simulink model "CW1_Pure_Pursuit_sim"  (R2023a)
settings: Solver=VariableStepAuto  StartTime=0.0  StopTime=Ts  RelTol=1e-3
values from neighbouring files (symbols this model uses):
  L = 3    [CW1_Pure_Pursuit.m]
  ld = 5    [CW1_Pure_Pursuit.m]
  psi_o = 90*rand(1)    [CW1_Pure_Pursuit.m]
  veh_v0 = 8    [CW1_Pure_Pursuit.m]    (also in DrivingScenario_LearnVersion.m)
  X_o = refPose(1,1)    [CW1_Pure_Pursuit.m]
  xRef = refPose(1,:)'    [CW1_Pure_Pursuit.m]
  Y_o = refPose(1,2)    [CW1_Pure_Pursuit.m]
  yRef = refPose(2,:)'    [CW1_Pure_Pursuit.m]
libraries: robotalgslib x1, autolibshared x1
settings Model: Creator=Gabriel  LastModifiedBy=Gabriel

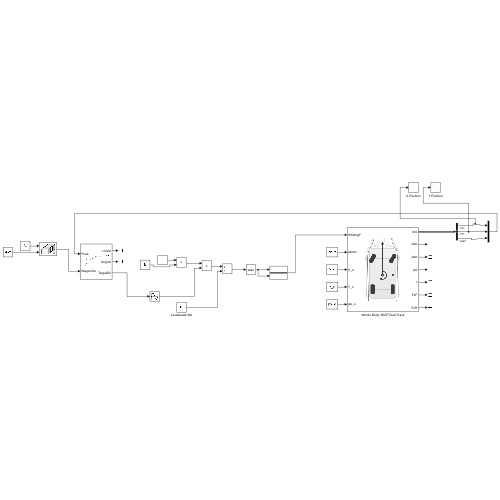
[thumbnail: Simulink's stored preview of the top-level diagram]
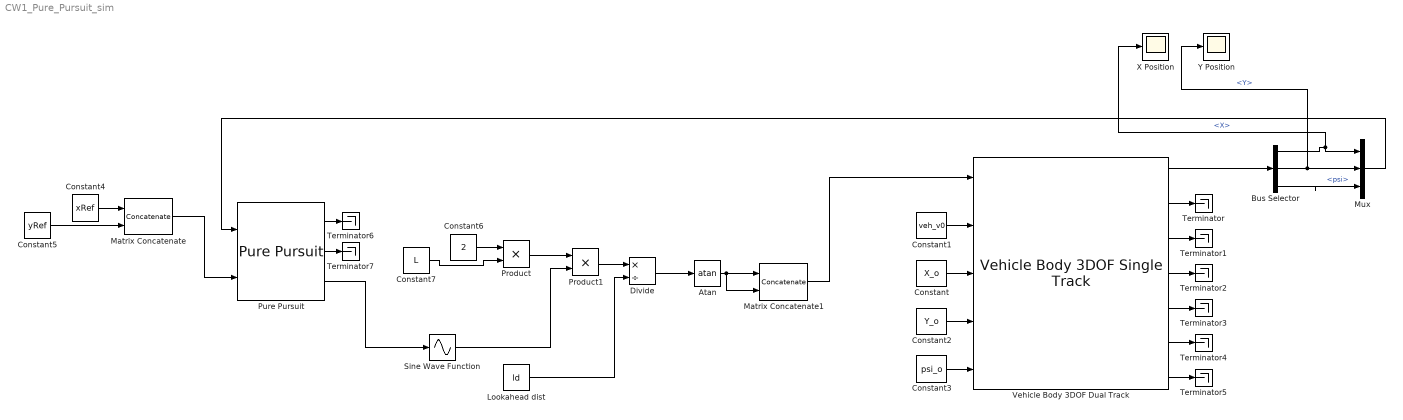
== system CW1_Pure_Pursuit_sim ==
  Atan : Trigonometry  Operator=atan
  Bus Selector : BusSelector  OutputSignals=InertFrm.Cg.Disp.X,InertFrm.Cg.Disp.Y,InertFrm.Cg.Ang.psi
  Constant : Constant  Value=X_o
  Constant1 : Constant  Value=veh_v0
  Constant2 : Constant  Value=Y_o
  Constant3 : Constant  Value=psi_o
  Constant4 : Constant  Value=xRef
  Constant5 : Constant  Value=yRef
  Constant6 : Constant  Value=2
  Constant7 : Constant  Value=L
  Divide : Product  Inputs=*/
  Lookahead dist : Constant  Value=ld
  Matrix Concatenate : Concatenate  Mode=Multidimensional array  ConcatenateDimension=2
  Matrix Concatenate1 : Concatenate  ConcatenateDimension=2
  Mux : Mux  Inputs=3
  Product : Product
  Product1 : Product
  Pure Pursuit : robotalgslib/Pure Pursuit  DesiredLinearVelocity=0.1  MaxAngularVelocity=1.0  LookaheadDistance=ld  TargetDirPort=on  SimulateUsing=Code generation
      settings: LibrarySourceBlock=navlib/Control Algorithms/Pure Pursuit
  Sine Wave Function : Sin  TimeSource=Use external signal  SampleTime=0
  Terminator{,1..7} (8 alike) : Terminator
  Vehicle Body 3DOF Dual Track : autolibshared/Vehicle Body 3DOF Single Track  trackMode=Dual  inputMode=External longitudinal velocity  frontSteerMode=on  rearSteerMode=off  windMode=off  muMode=off  extFMode=off  extMMode=off  htchFMode=off  htchMMode=off  extXo=on  extpsio=on  extxdoto=off  extro=off  extYo=on  extTamb=off  extydoto=off  aMode=2  NF=2  NR=2  m=2000  a=1.4  b=1.6  h=0.35  dh=1  hh=0.2  X_o=0  xdot_o=0  CalphaMode=off  sigmaMode=on  d=0  hl=0  w=[1.4,1.4]  Cy_f=12e3  Cy_r=11e3  sigma_f=.1  sigma_r=.1  alpha_f_brk=[-.1 .1]  Cy_f_data=[-9e3 9e3]  alpha_r_brk=[-.1 .1]  Cy_r_data=[-9e3 9e3]  Y_o=0  ydot_o=0  Izz=4000  psi_o=0  r_o=0  Af=2  Cd=.3  Cl=.1  Cpm=.1  beta_w=[0 0.01:0.01:0.3]  Cs=[0:0.03:0.9]  Cym=[0 1e-6:0.01:0.3]  Pabs=101325  Tair=273  g=9.81  mu=1  xdot_tol=.01  Fznom=5000  Fxtire_sat=7e4  Fytire_sat=7e4  longOff=0  latOff=0  vertOff=0  wrapAng=off
      settings: LibrarySourceBlock=vehdynlibeom/Vehicle Body 3DOF Dual Track
  X Position : Scope
  Y Position : Scope
  wires:
  Constant1/1 -> Vehicle Body 3DOF Dual Track/2
  Constant/1 -> Vehicle Body 3DOF Dual Track/3
  Constant2/1 -> Vehicle Body 3DOF Dual Track/4
  Constant3/1 -> Vehicle Body 3DOF Dual Track/5
  Constant4/1 -> Matrix Concatenate/1
  Constant5/1 -> Matrix Concatenate/2
  Matrix Concatenate/1 -> Pure Pursuit/2
  Vehicle Body 3DOF Dual Track/1 -> Bus Selector/1
  Bus Selector/1 -> X Position/1, Mux/1  "<X>"
  Bus Selector/2 -> Y Position/1, Mux/2  "<Y>"
  Bus Selector/3 -> Mux/3  "<psi>"
  Mux/1 -> Pure Pursuit/1
  Constant6/1 -> Product/1
  Constant7/1 -> Product/2
  Product/1 -> Product1/1
  Pure Pursuit/3 -> Sine Wave Function/1
  Sine Wave Function/1 -> Product1/2
  Product1/1 -> Divide/1
  Lookahead dist/1 -> Divide/2
  Divide/1 -> Atan/1
  Atan/1 -> Matrix Concatenate1/2, Matrix Concatenate1/1
  Matrix Concatenate1/1 -> Vehicle Body 3DOF Dual Track/1
  Vehicle Body 3DOF Dual Track/2 -> Terminator/1
  Vehicle Body 3DOF Dual Track/3 -> Terminator1/1
  Vehicle Body 3DOF Dual Track/4 -> Terminator2/1
  Vehicle Body 3DOF Dual Track/5 -> Terminator3/1
  Vehicle Body 3DOF Dual Track/6 -> Terminator4/1
  Vehicle Body 3DOF Dual Track/7 -> Terminator5/1
  Pure Pursuit/1 -> Terminator6/1
  Pure Pursuit/2 -> Terminator7/1
